simulink model "ControleFF_D_NL"  (R2020b)
settings: Solver=FixedStepAuto  StartTime=0  StopTime=10  FixedStep=1e-3  RelTol=1e-3
values from neighbouring files (symbols this model uses):
  alpha = alpha_vec(l)    [kermani_parameters.m]    (also in teste_controle_nao_linear.m = 1.25)
  Beff = 1    [kermani_parameters.m]    (also in teste_controle_nao_linear.m = 50)
  Fc = Fc_vec(k)    [kermani_parameters.m]    (also in teste_controle_nao_linear.m = 2173.5)
  Fs = Fs_vec(j)    [kermani_parameters.m]    (also in teste_controle_nao_linear.m = 2673.5)
  Jeff = 0.5    [kermani_parameters.m]    (also in teste_controle_nao_linear.m)
  K = (90/12)*(2*pi/60)    (= 0.785398163397)    [kermani_parameters.m]    (also in teste_controle_nao_linear.m)
  Kd = (2*xi*wn*Jeff - Beff)/K    (= 17.8253536263)    [kermani_parameters.m]    (also in teste_controle_nao_linear.m = -44.5633840657)
  Kp = (wn^2*Jeff)/K    (= 143.239448783)    [kermani_parameters.m]    (also in teste_controle_nao_linear.m)
  N = 3    [kermani_parameters.m]    (also in teste_controle_nao_linear.m)
  phi = 43.47    [teste_controle_nao_linear.m]
  r = 1./[231.22*4 139.138 139.138 231.22 231.22]    [kermani_parameters.m]    (also in teste_controle_nao_linear.m)
  sigma0 = sigma0_vec(m)    [kermani_parameters.m]    (also in teste_controle_nao_linear.m = 10000)
  sigma1 = sigma1_vec(n)    [kermani_parameters.m]    (also in teste_controle_nao_linear.m = 1000)
  sigma2 = sigma2_vec(o)    [kermani_parameters.m]    (also in teste_controle_nao_linear.m = 10)
libraries: simulink_extras x21
(part 8 of 14)

== matlab function ControleFF_D_NL/Compensador Feedforward2/Perturbação_d/MATLAB Function3 ==
  data: M input; V input; tau1 output; G input; ddTh input
function tau1  = calcul_dk1(M, V, G, ddTh)

tau1 = M(1,2)*ddTh(2) + M(1,3)*ddTh(3) + M(1,4)*ddTh(4) + M(1,5)*ddTh(5) ...
       + V(1) + G(1);

== matlab function ControleFF_D_NL/Compensador Feedforward2/Perturbação_d/MATLAB Function4 ==
  data: M input; V input; tau2 output; G input; ddTh input
function tau2  = calcul_dk2(M, V, G, ddTh)

tau2 = M(2,1)*ddTh(1) + M(2,3)*ddTh(3) + M(2,4)*ddTh(4) + M(2,5)*ddTh(5) ...
       + V(2) + G(2);

== matlab function ControleFF_D_NL/Compensador Feedforward1/Perturbação_d/MATLAB Function4 ==
  data: M input; V input; tau2 output; G input; ddTh input
function tau2  = calcul_dk2(M, V, G, ddTh)

tau2 = M(2,1)*ddTh(1) + M(2,3)*ddTh(3) + M(2,4)*ddTh(4) + M(2,5)*ddTh(5) ...
       + V(2) + G(2);

== matlab function ControleFF_D_NL/Compensador Feedforward2/Perturbação_d/MATLAB Function5 ==
  data: M input; V input; tau3 output; G input; ddTh input
function tau3  = calcul_dk3(M, V, G, ddTh)

tau3 = M(3,1)*ddTh(1) + M(3,2)*ddTh(2) + M(3,4)*ddTh(4) + M(3,5)*ddTh(5) ...
       + V(3) + G(3);

== matlab function ControleFF_D_NL/Compensador Feedforward2/Perturbação_d/MATLAB Function6 ==
  data: M input; V input; tau4 output; G input; ddTh input
function tau4 = calcul_dk4(M, V, G, ddTh)

tau4 = M(4,1)*ddTh(1) + M(4,2)*ddTh(2) + M(4,3)*ddTh(3) + M(4,5)*ddTh(5) ...
       + V(4) + G(4);

== matlab function ControleFF_D_NL/Compensador Feedforward2/Perturbação_d/MATLAB Function7 ==
  data: M input; V input; tau5 output; G input; ddTh input
function tau5  = calcul_dk5(M, V, G, ddTh)

tau5 = M(5,1)*ddTh(1) + M(5,2)*ddTh(2) + M(5,3)*ddTh(3) + M(5,4)*ddTh(4) ...
       + V(5) + G(5);

== matlab function ControleFF_D_NL/Compensador Feedforward2/Perturbação_d/MATLAB Function8 ==
  data: Th input; M output
function M = calcul_M(Th)

th1 = Th(1);
th2 = Th(2);
th3 = Th(3);
th4 = Th(4);
th5 = Th(5);

M = [ (87*cos(th2)^2*cos(th5))/2500 + (87*cos(th3)^2*cos(th5))/2500 - (33*cos(th2)^2*sin(th3))/50 + (53231*cos(th2)^2)/62500 + (8453*cos(th3)^2)/31250 - (9*cos(th5)^2)/3200 - (8453*cos(th2)^2*cos(th3)^2)/15625 - (217*cos(th2)^2*cos(th4)^2)/80000 + (9*cos(th2)^2*cos(th5)^2)/3200 - (217*cos(th3)^2*cos(th4)^2)/80000 + (9*cos(th3)^2*cos(th5)^2)/3200 - (87*cos(th2)^2*cos(th3)^2*cos(th5))/1250 - (33*cos(th2)*cos(th3)*sin(th2))/50 + (217*cos(th2)^2*cos(th3)^2*cos(th4)^2)/40000 - (9*cos(th2)^2*cos(th3)^2*cos(th5)^2)/1600 + (9*cos(th2)^2*cos(th4)^2*cos(th5)^2)/3200 + (9*cos(th3)^2*cos(th4)^2*cos(th5)^2)/3200 - (3*cos(th2)^2*cos(th5)*sin(th3))/80 - (9*cos(th2)^2*cos(th3)^2*cos(th4)^2*cos(th5)^2)/1600 - (3*cos(th2)*cos(th3)*cos(th5)*sin(th2))/80 + (8453*cos(th2)*cos(th3)*sin(th2)*sin(th3))/15625 - (87*cos(th2)*cos(th4)*sin(th2)*sin(th5))/2500 - (87*cos(th3)*cos(th4)*sin(th3)*sin(th5))/2500 - (3*cos(th2)^2*cos(th3)*cos(th4)*sin(th5))/80 + (3*cos(th2)*cos(th4)*sin(th2)*sin(th3)*sin(th5))/80 - (217*cos(th2)*cos(th3)*cos(th4)^2*sin(th2)*sin(th3))/40000 + (9*cos(th2)*cos(th3)*cos(th5)^2*sin(th2)*sin(th3))/1600 + (87*cos(th2)*cos(th3)^2*cos(th4)*sin(th2)*sin(th5))/1250 + (87*cos(th2)^2*cos(th3)*cos(th4)*sin(th3)*sin(th5))/1250 + (87*cos(th2)*cos(th3)*cos(th5)*sin(th2)*sin(th3))/1250 - (9*cos(th2)*cos(th4)*cos(th5)*sin(th2)*sin(th5))/1600 - (9*cos(th3)*cos(th4)*cos(th5)*sin(th3)*sin(th5))/1600 + (9*cos(th2)*cos(th3)*cos(th4)^2*cos(th5)^2*sin(th2)*sin(th3))/1600 + (9*cos(th2)*cos(th3)^2*cos(th4)*cos(th5)*sin(th2)*sin(th5))/800 + (9*cos(th2)^2*cos(th3)*cos(th4)*cos(th5)*sin(th3)*sin(th5))/800 + 3793/80000, -(sin(th4)*(1500*sin(th2)*sin(th5) - 217*cos(th2)*cos(th4)*sin(th3) - 217*cos(th3)*cos(th4)*sin(th2) + 1392*cos(th2)*cos(th3)*sin(th5) - 1392*sin(th2)*sin(th3)*sin(th5) + 225*cos(th2)*cos(th3)*cos(th5)*sin(th5) - 225*cos(th5)*sin(th2)*sin(th3)*sin(th5) + 225*cos(th2)*cos(th4)*cos(th5)^2*sin(th3) + 225*cos(th3)*cos(th4)*cos(th5)^2*sin(th2)))/80000, (sin(th4)*(217*cos(th2)*cos(th4)*sin(th3) + 217*cos(th3)*cos(th4)*sin(th2) - 1392*cos(th2)*cos(th3)*sin(th5) + 1392*sin(th2)*sin(th3)*sin(th5) - 225*cos(th2)*cos(th3)*cos(th5)*sin(th5) + 225*cos(th5)*sin(th2)*sin(th3)*sin(th5) - 225*cos(th2)*cos(th4)*cos(th5)^2*sin(th3) - 225*cos(th3)*cos(th4)*cos(th5)^2*sin(th2)))/80000, (489*cos(th2)*cos(th3))/80000 - (489*sin(th2)*sin(th3))/80000 - (3*cos(th2)*cos(th4)*sin(th5))/160 - (9*cos(th2)*cos(th3)*cos(th5)^2)/3200 + (9*cos(th5)^2*sin(th2)*sin(th3))/3200 + (87*cos(th2)*cos(th4)*sin(th3)*sin(th5))/5000 + (87*cos(th3)*cos(th4)*sin(th2)*sin(th5))/5000 + (9*cos(th2)*cos(th4)*cos(th5)*sin(th3)*sin(th5))/3200 + (9*cos(th3)*cos(th4)*cos(th5)*sin(th2)*sin(th5))/3200, (sin(th4)*(353*cos(th2)*sin(th3) + 353*cos(th3)*sin(th2) - 1500*cos(th2)*cos(th5) + 1392*cos(th2)*cos(th5)*sin(th3) + 1392*cos(th3)*cos(th5)*sin(th2)))/80000;
                                                                                                                                                                                                                                                                                                                                                                                                                                                                                                                                                                                                                                                                                                                                                                                                                                                                                                                                                                                                                                                                                                                                                                                                                                                                                                                                                                                                                                                                                                                                                                                            -(sin(th4)*(1500*sin(th2)*sin(th5) - 217*cos(th2)*cos(th4)*sin(th3) - 217*cos(th3)*cos(th4)*sin(th2) + 1392*cos(th2)*cos(th3)*sin(th5) - 1392*sin(th2)*sin(th3)*sin(th5) + 225*cos(th2)*cos(th3)*cos(th5)*sin(th5) - 225*cos(th5)*sin(th2)*sin(th3)*sin(th5) + 225*cos(th2)*cos(th4)*cos(th5)^2*sin(th3) + 225*cos(th3)*cos(th4)*cos(th5)^2*sin(th2)))/80000,                                                                                                                                                                                                                       (87*cos(th5))/2500 - (33*sin(th3))/50 - (3*cos(th5)*sin(th3))/80 + (217*cos(th4)^2)/80000 + (9*cos(th5)^2)/3200 - (9*cos(th4)^2*cos(th5)^2)/3200 - (3*cos(th3)*cos(th4)*sin(th5))/80 + 54781/62500,                                                                                                                                                                                   (87*cos(th5))/2500 - (33*sin(th3))/100 - (3*cos(th5)*sin(th3))/160 + (217*cos(th4)^2)/80000 + (9*cos(th5)^2)/3200 - (9*cos(th4)^2*cos(th5)^2)/3200 - (3*cos(th3)*cos(th4)*sin(th5))/160 + 72749/250000,                                                                                                                                                                                                                                                                                                                                                                                                                     -(3*sin(th4)*sin(th5)*(75*cos(th5) - 500*sin(th3) + 464))/80000,                                                          (353*cos(th4))/80000 - (3*cos(th3)*sin(th5))/160 + (87*cos(th4)*cos(th5))/5000 - (3*cos(th4)*cos(th5)*sin(th3))/160;
                                                                                                                                                                                                                                                                                                                                                                                                                                                                                                                                                                                                                                                                                                                                                                                                                                                                                                                                                                                                                                                                                                                                                                                                                                                                                                                                                                                                                                                                                                                                                                                                                            (sin(th4)*(217*cos(th2)*cos(th4)*sin(th3) + 217*cos(th3)*cos(th4)*sin(th2) - 1392*cos(th2)*cos(th3)*sin(th5) + 1392*sin(th2)*sin(th3)*sin(th5) - 225*cos(th2)*cos(th3)*cos(th5)*sin(th5) + 225*cos(th5)*sin(th2)*sin(th3)*sin(th5) - 225*cos(th2)*cos(th4)*cos(th5)^2*sin(th3) - 225*cos(th3)*cos(th4)*cos(th5)^2*sin(th2)))/80000,                                                                                                                                                                                                                   (87*cos(th5))/2500 - (33*sin(th3))/100 - (3*cos(th5)*sin(th3))/160 + (217*cos(th4)^2)/80000 + (9*cos(th5)^2)/3200 - (9*cos(th4)^2*cos(th5)^2)/3200 - (3*cos(th3)*cos(th4)*sin(th5))/160 + 72749/250000,                                                                                                                                                                                                                                                                                          (87*cos(th5))/2500 + (217*cos(th4)^2)/80000 + (9*cos(th5)^2)/3200 - (9*cos(th4)^2*cos(th5)^2)/3200 + 72749/250000,                                                                                                                                                                                                                                                                                                                                                                                                                                       -(3*sin(th4)*sin(th5)*(75*cos(th5) + 464))/80000,                                                                                                                                                         (cos(th4)*(1392*cos(th5) + 353))/80000;
                                                                                                                                                                                                                                                                                                                                                                                                                                                                                                                                                                                                                                                                                                                                                                                                                                                                                                                                                                                                                                                                                                                                                                                                                                                                                                                                                                                                                                                                                                                                                      (489*cos(th2)*cos(th3))/80000 - (489*sin(th2)*sin(th3))/80000 - (3*cos(th2)*cos(th4)*sin(th5))/160 - (9*cos(th2)*cos(th3)*cos(th5)^2)/3200 + (9*cos(th5)^2*sin(th2)*sin(th3))/3200 + (87*cos(th2)*cos(th4)*sin(th3)*sin(th5))/5000 + (87*cos(th3)*cos(th4)*sin(th2)*sin(th5))/5000 + (9*cos(th2)*cos(th4)*cos(th5)*sin(th3)*sin(th5))/3200 + (9*cos(th3)*cos(th4)*cos(th5)*sin(th2)*sin(th5))/3200,                                                                                                                                                                                                                                                                                                                                                                               -(3*sin(th4)*sin(th5)*(75*cos(th5) - 500*sin(th3) + 464))/80000,                                                                                                                                                                                                                                                                                                                                                                 -(3*sin(th4)*sin(th5)*(75*cos(th5) + 464))/80000,                                                                                                                                                                                                                                                                                                                                                                                                                                                              489/80000 - (9*cos(th5)^2)/3200,                                                                                                                                                                                                    0;
                                                                                                                                                                                                                                                                                                                                                                                                                                                                                                                                                                                                                                                                                                                                                                                                                                                                                                                                                                                                                                                                                                                                                                                                                                                                                                                                                                                                                                                                                                                                                                                                                                                                                                                                                                                                                                                 (sin(th4)*(353*cos(th2)*sin(th3) + 353*cos(th3)*sin(th2) - 1500*cos(th2)*cos(th5) + 1392*cos(th2)*cos(th5)*sin(th3) + 1392*cos(th3)*cos(th5)*sin(th2)))/80000,                                                                                                                                                                                                                                                                                                               (353*cos(th4))/80000 - (3*cos(th3)*sin(th5))/160 + (87*cos(th4)*cos(th5))/5000 - (3*cos(th4)*cos(th5)*sin(th3))/160,                                                                                                                                                                                                                                                                                                                                                                              (cos(th4)*(1392*cos(th5) + 353))/80000,                                                                                                                                                                                                                                                                                                                                                                                                                                                                                               0,                                                                                                                                                                                            353/80000];

== matlab function ControleFF_D_NL/Compensador Feedforward2/Perturbação_d/MATLAB Function9 ==
  data: Th input; G output
function G = calcul_G(Th)

g = 9.80665;
th1 = Th(1);
th2 = Th(2);
th3 = Th(3);
th4 = Th(4);
th5 = Th(5);

G = [                                                                                                                                                                                                                                                                                               0;
 -g*((49*cos(th2)*sin(th3))/125 - cos(th2)/2 + (49*cos(th3)*sin(th2))/125 + (3*cos(th2)*cos(th5)*sin(th3))/40 + (3*cos(th3)*cos(th5)*sin(th2))/40 + (3*cos(th2)*cos(th3)*cos(th4)*sin(th5))/40 - (3*cos(th4)*sin(th2)*sin(th3)*sin(th5))/40);
                 -g*((49*cos(th2)*sin(th3))/125 + (49*cos(th3)*sin(th2))/125 + (3*cos(th2)*cos(th5)*sin(th3))/40 + (3*cos(th3)*cos(th5)*sin(th2))/40 + (3*cos(th2)*cos(th3)*cos(th4)*sin(th5))/40 - (3*cos(th4)*sin(th2)*sin(th3)*sin(th5))/40);
                                                                                                                                                                                                                                                (3*g*sin(th4)*sin(th5)*sin(th2 + th3))/40;
                                                                                       -g*((3*cos(th2)*cos(th3)*sin(th5))/40 - (3*sin(th2)*sin(th3)*sin(th5))/40 + (3*cos(th2)*cos(th4)*cos(th5)*sin(th3))/40 + (3*cos(th3)*cos(th4)*cos(th5)*sin(th2))/40)];
